simulink model "I_and_I"  (R2020a)
settings: Solver=VariableStepAuto  StartTime=0.0  StopTime=100  RelTol=1e-3
InitFcn:
  | varSym
values from neighbouring files (symbols this model uses):
  a1 = 1    [varSym.m]
  a2 = 1    [varSym.m]
  ad1 = 0.1    [varSym.m]
  est0 = [0;0]    [varSym.m]
  md2 = 0    [varSym.m]
  vd2 = 0.01    [varSym.m]
  w1 = 100    [varSym.m]
  w2 = 1    [varSym.m]
  wChange = 0.01    [varSym.m]
  wd1 = 50    [varSym.m]
  wMax = 1    [varSym.m]
libraries: simulink x1
settings Model: Creator=alfystar  LastModifiedBy=gabriele

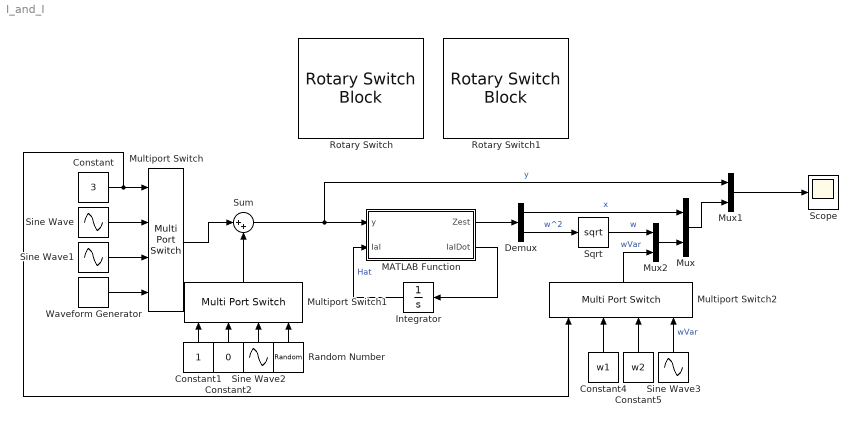
== system I_and_I ==
  Constant : Constant  Value=3
  Constant1 : Constant
  Constant2 : Constant  Value=0
  Constant4 : Constant  Value=w1
  Constant5 : Constant  Value=w2
  Demux : Demux  Outputs=2
  Integrator : Integrator  InitialCondition=est0
  MATLAB Function : MATLAB Function  TreatAsAtomicUnit=on
  Multiport Switch : MultiPortSwitch
  Multiport Switch1 : MultiPortSwitch
  Multiport Switch2 : MultiPortSwitch
  Mux : Mux  Inputs=2
  Mux1 : Mux  Inputs=2
  Mux2 : Mux  Inputs=2
  Random Number : RandomNumber  Mean=md2  Variance=vd2  SampleTime=0.1
  Rotary Switch : RotarySwitchBlock  LabelPosition=Hide
      settings: Values={{'y1', 'y2', 'varFreq'}, [1 2 3]}
  Rotary Switch1 : RotarySwitchBlock  LabelPosition=Hide
      settings: Values={{'Off', 'Sin', 'Ran'}, [1 2 3]}
  Scope : Scope
  Sine Wave : Sin  Amplitude=a1  Frequency=w1  SampleTime=0
  Sine Wave1 : Sin  Amplitude=a2  Frequency=w2  SampleTime=0
  Sine Wave2 : Sin  Amplitude=ad1  Frequency=wd1  SampleTime=0
  Sine Wave3 : Sin  Amplitude=wMax  Bias=wMax+0.01  Frequency=wChange  SampleTime=0
  Sqrt : Sqrt  SaturateOnIntegerOverflow=on
  Sum : Sum  Inputs=|++
  Waveform Generator : simulink/Sources/Waveform Generator  OutMin=[]  OutMax=[]  OutDataTypeStr=double  SelectedSignal=1  Signals=sin('Amplitude', 1, 'Frequency', sin(wMax,wChange,0)+wMax+0.01, 'Phase', 0)  BlockNames=MultiportSwitch_ca3327b5d59143e  SampleTime=0.1
  wires:
  Sine Wave1/1 -> Multiport Switch/3
  Sine Wave/1 -> Multiport Switch/2
  Sine Wave2/1 -> Multiport Switch1/3
  Constant2/1 -> Multiport Switch1/2
  Constant1/1 -> Multiport Switch1/1
  Random Number/1 -> Multiport Switch1/4
  Multiport Switch/1 -> Sum/1
  Multiport Switch1/1 -> Sum/2
  Sum/1 -> Mux1/1, MATLAB Function/1(y)  "y"
  MATLAB Function/2(IaIDot) -> Integrator/1
  Integrator/1 -> MATLAB Function/2(IaI)  "Hat"
  Demux/1 -> Mux/1  "x"
  Demux/2 -> Sqrt/1  "w^2"
  MATLAB Function/1(Zest) -> Demux/1
  Mux/1 -> Mux1/2
  Sqrt/1 -> Mux2/1  "w"
  Mux1/1 -> Scope/1
  Waveform Generator/1 -> Multiport Switch/4
  Mux2/1 -> Mux/2
  Multiport Switch2/1 -> Mux2/2  "wVar"
  Sine Wave3/1 -> Multiport Switch2/4  "wVar"
  Constant/1 -> Multiport Switch/1, Multiport Switch2/1
  Constant5/1 -> Multiport Switch2/3
  Constant4/1 -> Multiport Switch2/2

== matlab function I_and_I/MATLAB Function ==
  data: Zest output; y input; IaIDot output; IaI input
function [Zest, IaIDot] = IandI(y,IaI)
%       |x2Hat   |           |x2HatDot   |
% IaI = |        |  IaIDot = |           |
%       |tethaHat|           |tethaHatDot|

%        |x2Est   |
% Zest = |        |
%        |tethaEst|

coder.extrinsic('evalin', 'assignin')
k1 = 0;                  
k1 = evalin('base','k1');


Zest=zeros(2,1);
Zest(2) = y*IaI(1) + IaI(2);
Zest(1) = k1*y + IaI(1)*(k1^2+Zest(2));

IaIDot=zeros(2,1);

x2HatDot = -k1*IaI(1)-y;
thetaHatDot = -(k1*y*IaI(1) + k1^2*IaI(1)^2 +...
    y*x2HatDot + y*IaI(1)^3 + IaI(2)*IaI(1)^2);

IaIDot(1) = x2HatDot;
IaIDot(2) = thetaHatDot;
% IaIDot(1) = -k1*IaI(1) + (k1^2+Zest(2))*y;
% 
% IaIDot(2) = -k1*y*IaI(1) - IaI(2)*Zest(1)^2 + 0;

end
